simulink model "LinearSimulinkModel"  (Simulink 7.7)
settings: Solver=ode45  StartTime=0.0  StopTime=60.0  RelTol=1e-6
values from neighbouring files (symbols this model uses):
  ba = 6.5E-6    (= 6.5e-06)    [LinearPrelim.m]
  bt = btavg    (= 2.97258e-05)    [LinearPrelim.m]
  DenB = [(C5*C1-C3*C3), (C1*btavg+C5*ba), (ba*btavg-C4*C5), (-C4*btavg), 0]    [LinearPrelim.m]
  g = 9.81    [LinearPrelim.m]
  I1zt = 6.78e-4 + 3.50514e-5    (= 0.0007130514)    [LinearPrelim.m]
  Ix2 = 8.1e-6    (= 8.1e-06)    [LinearPrelim.m]
  Ixz2 = 2.03e-5    (= 2.03e-05)    [LinearPrelim.m]
  Iy2 = 3.711e-4    (= 0.0003711)    [LinearPrelim.m]
  Iz2 = 3.646e-4    (= 0.0003646)    [LinearPrelim.m]
  Ka = 1    [LinearPrelim.m]
  Kt = 0.0314499    [LinearPrelim.m]
  l1 = 0.10825640    (= 0.1082564)    [LinearPrelim.m]
  l2c = 0.0856786    [LinearPrelim.m]
  m2 = 0.0820142    [LinearPrelim.m]
  NumBA = [-C3, 0, 0]    [LinearPrelim.m]
  NumBT = [C1, ba, -C4]    [LinearPrelim.m]
undefined symbols (not defined in the file or in its folder): DenAC, DenTC, NumAC, NumTC
libraries: simulink_extras x2
settings Model: Creator=jrpeterson  LastModifiedBy=jrpeterson
settings HardwareCC: ProdBitPerInt=16  ProdBitPerPointer=8  ProdIntDivRoundTo=Zero  ProdWordSize=8  ProdShiftRightIntArith=off  ProdHWDeviceType=Intel->8051 Compatible

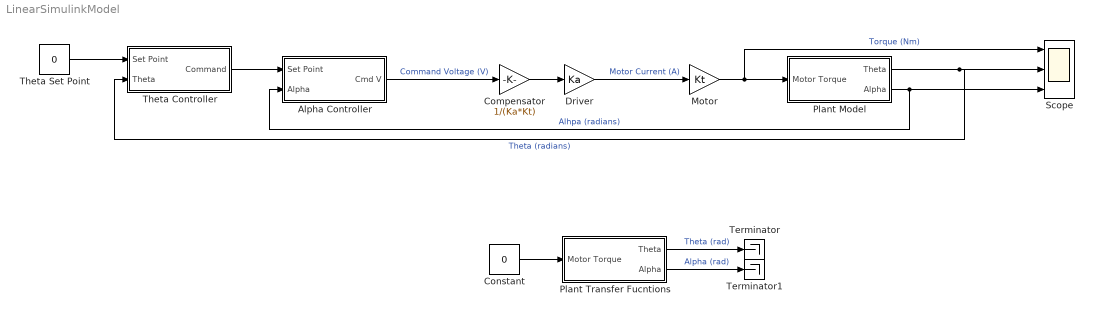
== system LinearSimulinkModel ==
  Alpha Controller : Subsystem
  Compensator : Gain  Gain=1/(Ka*Kt)
  Constant : Constant  Value=0
  Driver : Gain  Gain=Ka
  "Motor " : Gain  Gain=Kt
  Plant Model : Subsystem
  Plant Transfer Fucntions : Subsystem
  Scope : Scope  NumInputPorts=3
      settings: YMin=-5~-5~-5  YMax=5~5~5
  Terminator : Terminator
  Terminator1 : Terminator
  Theta Controller : Subsystem
  Theta Set Point : Constant  Value=0
  wires:
  "Motor "/1 -> Scope/1, Plant Model/1(Motor Torque)  "Torque (Nm)"
  Driver/1 -> "Motor "/1  "Motor Current (A)"
  Alpha Controller/1(Cmd V) -> Compensator/1  "Command Voltage (V)"
  Compensator/1 -> Driver/1
  Theta Set Point/1 -> Theta Controller/1(Set Point)
  Theta Controller/1(Command) -> Alpha Controller/1(Set Point)
  Plant Model/1(Theta) -> Scope/2, Theta Controller/2(Theta)  "Theta (radians)"
  Plant Model/2(Alpha) -> Scope/3, Alpha Controller/2(Alpha)  "Alhpa (radians)"
  Plant Transfer Fucntions/1(Theta) -> Terminator/1  "Theta (rad)"
  Plant Transfer Fucntions/2(Alpha) -> Terminator1/1  "Alpha (rad)"
  Constant/1 -> Plant Transfer Fucntions/1(Motor Torque)

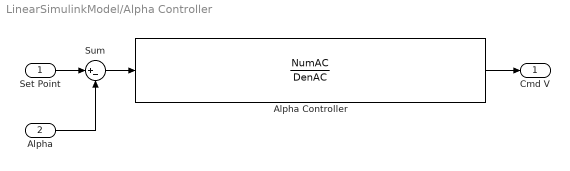
== system LinearSimulinkModel/Alpha Controller ==
  Set Point : Inport
  Alpha : Inport  Port=2
  Alpha Controller : TransferFcn  Numerator=NumAC  Denominator=DenAC
  Sum : Sum  Inputs=|+-
  Cmd V : Outport
  wires:
  Alpha Controller/1 -> Cmd V/1
  Set Point/1 -> Sum/1
  Alpha/1 -> Sum/2
  Sum/1 -> Alpha Controller/1

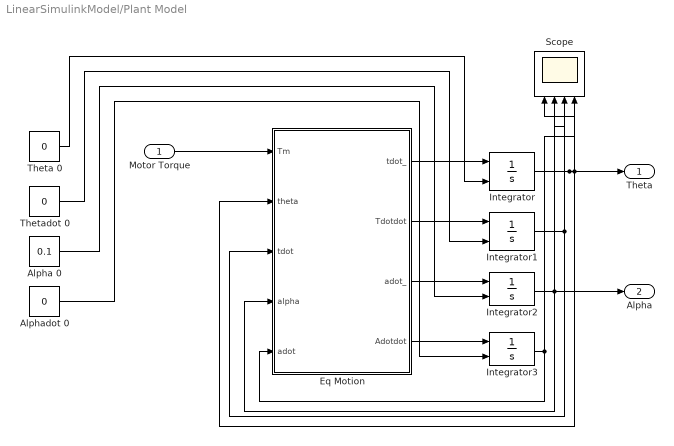
== system LinearSimulinkModel/Plant Model ==
  Motor Torque : Inport
  Alpha 0 : Constant  Value=0.1
  Alphadot 0 : Constant  Value=0
  Eq Motion : Stateflow chart  TreatAsAtomicUnit=on
  Integrator{,1..3} (4 alike) : Integrator  InitialConditionSource=external
  Scope : Scope  NumInputPorts=4
      settings: YMin=-5~-5~-5~-5  YMax=5~5~5~5  SaveName=LinearSystemResponse
  Theta 0 : Constant  Value=0
  Thetadot 0 : Constant  Value=0
  Theta : Outport
  Alpha : Outport  Port=2
  wires:
  Motor Torque/1 -> Eq Motion/1(Tm)
  Eq Motion/1(tdot_) -> Integrator/1
  Eq Motion/2(Tdotdot) -> Integrator1/1
  Eq Motion/3(adot_) -> Integrator2/1
  Eq Motion/4(Adotdot) -> Integrator3/1
  Integrator3/1 -> Eq Motion/5(adot), Scope/4
  Integrator2/1 -> Eq Motion/4(alpha), Alpha/1, Scope/3
  Integrator1/1 -> Eq Motion/3(tdot), Scope/2
  Integrator/1 -> Eq Motion/2(theta), Scope/1, Theta/1
  Theta 0/1 -> Integrator/2
  Thetadot 0/1 -> Integrator1/2
  Alpha 0/1 -> Integrator2/2
  Alphadot 0/1 -> Integrator3/2

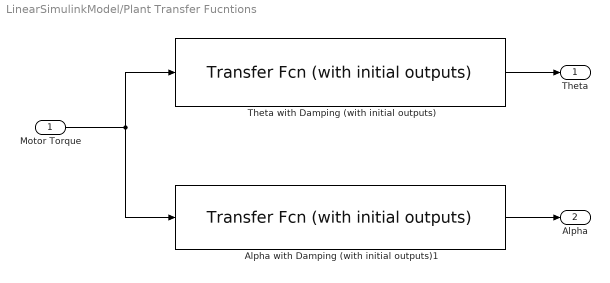
== system LinearSimulinkModel/Plant Transfer Fucntions ==
  Motor Torque : Inport
  Alpha with Damping (with initial outputs)1 : simulink_extras/Additional Linear/Transfer Fcn (with initial outputs)  SystemSampleTime=-1  N=NumBA  D=DenB  Y0=.1  U0=0
  Theta with Damping (with initial outputs) : simulink_extras/Additional Linear/Transfer Fcn (with initial outputs)  SystemSampleTime=-1  N=NumBT  D=DenB  Y0=0  U0=0
  Theta : Outport
  Alpha : Outport  Port=2
  wires:
  Alpha with Damping (with initial outputs)1/1 -> Alpha/1
  Motor Torque/1 -> Theta with Damping (with initial outputs)/1, Alpha with Damping (with initial outputs)1/1
  Theta with Damping (with initial outputs)/1 -> Theta/1

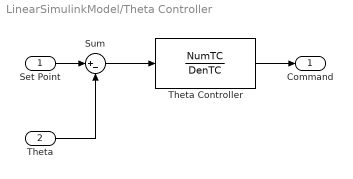
== system LinearSimulinkModel/Theta Controller ==
  Set Point : Inport
  Theta : Inport  Port=2
  Sum : Sum  Inputs=|+-
  Theta Controller : TransferFcn  Numerator=NumTC  Denominator=DenTC
  Command : Outport
  wires:
  Set Point/1 -> Sum/1
  Theta/1 -> Sum/2
  Sum/1 -> Theta Controller/1
  Theta Controller/1 -> Command/1

== matlab function Plant Model/Eq Motion ==
  data: Tm input double; tdot_ output double; theta input double; tdot input double; alpha input double; adot input double; m2 parameter double; I1zt parameter double; Ix2 parameter double; Iy2 parameter double; Iz2 parameter double; Ixz2 parameter double; g parameter double; l1 parameter double; l2c parameter double; ba parameter double; bt parameter double; Tdotdot output double; adot_ output double; Adotdot output double
function [tdot_, Tdotdot, adot_, Adotdot] = eqMotionLinear(Tm, theta,tdot,alpha,adot, m2, I1zt, Ix2, Iy2, Iz2, Ixz2, g, l1, l2c, ba, bt)
% we currently assume differential coulomb friction and damping for theta,
% but not for alpha
tdot_ = tdot;
adot_ = adot;

%%%%%%%%%%%%
% Linear Damping

% Neglect Friction

C1 = Iz2+m2*l2c*l2c;  C2 = Iy2+m2*l2c*l2c;   C3 = m2*l1*l2c-Ixz2;  C4 = l2c*m2*g;

C5 = I1zt + Ix2 + m2*l1*l1;  C6 = C5*C1-C3*C3;

Tdotdot = (1/C6)*(C3*ba*adot - C3*C4*alpha - C1*bt*tdot + C1*Tm);

Adotdot = (1/C6)*(-ba*adot*C5 + bt*tdot*C3 + alpha*C4*C5 - C3*Tm);
end
